simulink model "uncompensated_system"  (R2017a)
settings: Solver=FixedStepAuto  StartTime=0.0  StopTime=10.0  FixedStep=10^-3  RelTol=1e-3
settings Model: Creator=Sean  LastModifiedBy=Sean

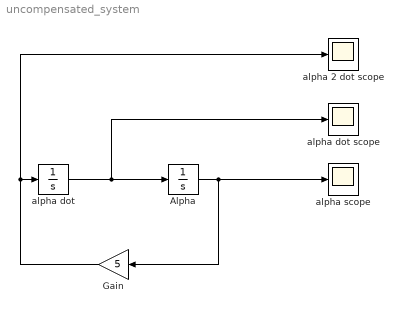
== system uncompensated_system ==
  Alpha : Integrator  InitialCondition=0.12
  Gain : Gain  Gain=5
  alpha 2 dot scope : Scope
  alpha dot : Integrator  InitialCondition=0.45
  alpha dot scope : Scope
  alpha scope : Scope
  wires:
  alpha dot/1 -> alpha dot scope/1, Alpha/1
  Alpha/1 -> alpha scope/1, Gain/1
  Gain/1 -> alpha 2 dot scope/1, alpha dot/1
